simulink model "specifications_artificial"  (R2019b)
settings: Solver=FixedStepAuto  StartTime=0.0  StopTime=10.0  FixedStep=fixedStepSize  RelTol=1e-3
settings Model: Creator=JEDDELAN  LastModifiedBy=jeddelan
settings DataIOCC: ReturnWorkspaceOutputs=off
settings DebuggingCC: ArithmeticOperatorsInVariantConditions=warning
settings SFSimCC: SimUseLocalCustomCode=off  CustomCodeUndefinedFunction=UseInterfaceOnly
settings RTWCC: RTWUseLocalCustomCode=off

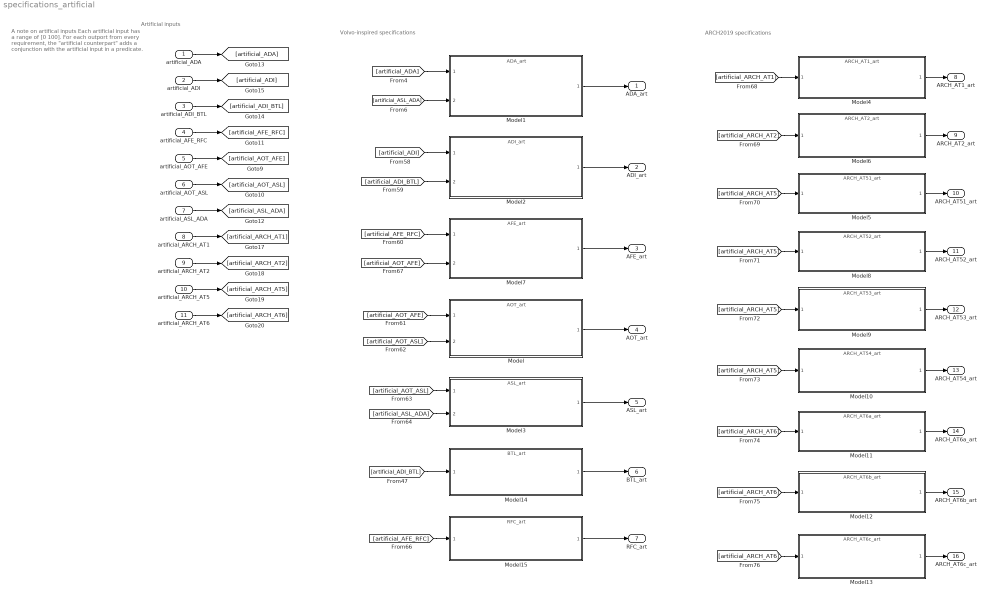
== system specifications_artificial ==
  note: A note on artifical inputs
      | Each artificial input has a range of [0 100].
      | For each outport from every requirement, the
      | "artificial counterpart" adds a conjunction with
      | the artificial input in a predicate.
  note: Artificial inputs
  note: ARCH2019 specifications
  note: Volvo-inspired specifications
  artificial_ADA : Inport
  artificial_ADI : Inport  Port=2
  artificial_ADI_BTL : Inport  Port=3
  artificial_AFE_RFC : Inport  Port=4
  artificial_AOT_AFE : Inport  Port=5
  artificial_AOT_ASL : Inport  Port=6
  artificial_ASL_ADA : Inport  Port=7
  artificial_ARCH_AT1 : Inport  Port=8
  artificial_ARCH_AT2 : Inport  Port=9
  artificial_ARCH_AT5 : Inport  Port=10
  artificial_ARCH_AT6 : Inport  Port=11
  Model : ModelReference  ModelNameDialog=AOT_art.slx  SimulationMode=Normal  ModelReferenceVersion=1.542
  Model1 : ModelReference  ModelNameDialog=ADA_art.slx  SimulationMode=Normal  ModelReferenceVersion=1.678
  Model10 : ModelReference  ModelNameDialog=ARCH_AT54_art.slx  SimulationMode=Normal  ModelReferenceVersion=1.499
  Model11 : ModelReference  ModelNameDialog=ARCH_AT6a_art.slx  SimulationMode=Normal  ModelReferenceVersion=1.506
  Model12 : ModelReference  ModelNameDialog=ARCH_AT6b_art.slx  SimulationMode=Normal  ModelReferenceVersion=1.507
  Model13 : ModelReference  ModelNameDialog=ARCH_AT6c_art.slx  SimulationMode=Normal  ModelReferenceVersion=1.504
  Model14 : ModelReference  ModelNameDialog=BTL_art.slx  SimulationMode=Normal  ModelReferenceVersion=1.2799
  Model15 : ModelReference  ModelNameDialog=RFC_art.slx  SimulationMode=Normal  ModelReferenceVersion=1.2718
  Model2 : ModelReference  ModelNameDialog=ADI_art.slx  SimulationMode=Normal  ModelReferenceVersion=1.400
  Model3 : ModelReference  ModelNameDialog=ASL_art.slx  SimulationMode=Normal  ModelReferenceVersion=1.532
  Model4 : ModelReference  ModelNameDialog=ARCH_AT1_art.slx  SimulationMode=Normal  ModelReferenceVersion=1.439
  Model5 : ModelReference  ModelNameDialog=ARCH_AT51_art.slx  SimulationMode=Normal  ModelReferenceVersion=1.499
  Model6 : ModelReference  ModelNameDialog=ARCH_AT2_art.slx  SimulationMode=Normal  ModelReferenceVersion=1.440
  Model7 : ModelReference  ModelNameDialog=AFE_art.slx  SimulationMode=Normal  ModelReferenceVersion=1.527
  Model8 : ModelReference  ModelNameDialog=ARCH_AT52_art.slx  SimulationMode=Normal  ModelReferenceVersion=1.501
  Model9 : ModelReference  ModelNameDialog=ARCH_AT53_art.slx  SimulationMode=Normal  ModelReferenceVersion=1.510
  ADA_art : Outport  VectorParamsAs1DForOutWhenUnconnected=off
  ADI_art : Outport  Port=2  VectorParamsAs1DForOutWhenUnconnected=off
  AFE_art : Outport  Port=3  VectorParamsAs1DForOutWhenUnconnected=off
  AOT_art : Outport  Port=4  VectorParamsAs1DForOutWhenUnconnected=off
  ASL_art : Outport  Port=5  VectorParamsAs1DForOutWhenUnconnected=off
  BTL_art : Outport  Port=6  VectorParamsAs1DForOutWhenUnconnected=off
  RFC_art : Outport  Port=7  VectorParamsAs1DForOutWhenUnconnected=off
  ARCH_AT1_art : Outport  Port=8  VectorParamsAs1DForOutWhenUnconnected=off
  ARCH_AT2_art : Outport  Port=9  VectorParamsAs1DForOutWhenUnconnected=off
  ARCH_AT51_art : Outport  Port=10  VectorParamsAs1DForOutWhenUnconnected=off
  ARCH_AT52_art : Outport  Port=11  VectorParamsAs1DForOutWhenUnconnected=off
  ARCH_AT53_art : Outport  Port=12  VectorParamsAs1DForOutWhenUnconnected=off
  ARCH_AT54_art : Outport  Port=13  VectorParamsAs1DForOutWhenUnconnected=off
  ARCH_AT6a_art : Outport  Port=14  VectorParamsAs1DForOutWhenUnconnected=off
  ARCH_AT6b_art : Outport  Port=15  VectorParamsAs1DForOutWhenUnconnected=off
  ARCH_AT6c_art : Outport  Port=16  VectorParamsAs1DForOutWhenUnconnected=off
  wires:
  Model/1 -> AOT_art/1
  [artificial_ASL_ADA] -> Model1/2
  [artificial_ADA] -> Model1/1
  Model1/1 -> ADA_art/1
  Model2/1 -> ADI_art/1
  Model3/1 -> ASL_art/1
  Model4/1 -> ARCH_AT1_art/1
  Model5/1 -> ARCH_AT51_art/1
  Model6/1 -> ARCH_AT2_art/1
  Model7/1 -> AFE_art/1
  Model8/1 -> ARCH_AT52_art/1
  Model9/1 -> ARCH_AT53_art/1
  Model10/1 -> ARCH_AT54_art/1
  Model11/1 -> ARCH_AT6a_art/1
  Model12/1 -> ARCH_AT6b_art/1
  Model13/1 -> ARCH_AT6c_art/1
  [artificial_ADI_BTL] -> Model14/1
  Model14/1 -> BTL_art/1
  Model15/1 -> RFC_art/1
  artificial_AOT_AFE/1 -> [artificial_AOT_AFE]
  artificial_AOT_ASL/1 -> [artificial_AOT_ASL]
  artificial_AFE_RFC/1 -> [artificial_AFE_RFC]
  artificial_ASL_ADA/1 -> [artificial_ASL_ADA]
  artificial_ADI_BTL/1 -> [artificial_ADI_BTL]
  artificial_ADI/1 -> [artificial_ADI]
  artificial_ARCH_AT6/1 -> [artificial_ARCH_AT6]
  artificial_ARCH_AT5/1 -> [artificial_ARCH_AT5]
  artificial_ARCH_AT2/1 -> [artificial_ARCH_AT2]
  artificial_ARCH_AT1/1 -> [artificial_ARCH_AT1]
  [artificial_ADI] -> Model2/1
  [artificial_ADI_BTL] -> Model2/2
  [artificial_AFE_RFC] -> Model7/1
  [artificial_AOT_AFE] -> Model/1
  [artificial_AOT_ASL] -> Model/2
  [artificial_AOT_ASL] -> Model3/1
  [artificial_ASL_ADA] -> Model3/2
  [artificial_AFE_RFC] -> Model15/1
  [artificial_AOT_AFE] -> Model7/2
  artificial_ADA/1 -> [artificial_ADA]
  [artificial_ARCH_AT1] -> Model4/1
  [artificial_ARCH_AT2] -> Model6/1
  [artificial_ARCH_AT5] -> Model5/1
  [artificial_ARCH_AT5] -> Model8/1
  [artificial_ARCH_AT5] -> Model9/1
  [artificial_ARCH_AT5] -> Model10/1
  [artificial_ARCH_AT6] -> Model11/1
  [artificial_ARCH_AT6] -> Model12/1
  [artificial_ARCH_AT6] -> Model13/1
